simulink model "stepchange_timevarying_change_pure_dual"  (R2022b)
settings: Solver=VariableStepAuto  StartTime=0.0  StopTime=8  MaxStep=0.001  RelTol=1e-3
values from neighbouring files (symbols this model uses):
  A = [eye(N),     -LoadZ^-1,   B; zeros(BN,N),  R_l^-1*B',   eye(BN); zeros(1,N),  zeros(1,N),   V_r'*B ]    [stepchange_timevarying_change_initial_document.m]
  A_r = kron(diag(r),eye(N+BN+1))    [stepchange_timevarying_change_initial_document.m]
  alpha_u = [1.1    1.4    1.8    1.1           1.1    1.9    1.9    1.2           1.3    1.4    1.8    0.6           1.8    2.1    1.5    0.9]'    [stepchange_timevarying_change_initial_document.m]
  alpha_V = [0.7    0.6    0.8    0.9           0.7    1.2    0.8    1.24           0.3    0.3    0.0    1.70           1.0    0.5    1.1    1.0]'    [stepchange_timevarying_change_initial_document.m]
  alpha_w = 0.8    [stepchange_timevarying_change_initial_document.m]
  BN = size(Line1,1)/2    [stepchange_timevarying_change_initial_document.m]
  box_gain = 100    [stepchange_timevarying_change_initial_document.m]
  changerate = 3    [stepchange_timevarying_change_initial_document.m]
  changetime = 5    [stepchange_timevarying_change_initial_document.m]
  changevariance = 0.1    [stepchange_timevarying_change_initial_document.m]
  constraint_gain = 200    [stepchange_timevarying_change_initial_document.m]
  Dw = 0.01    [stepchange_timevarying_change_initial_document.m]
  epsilon = 2    [stepchange_timevarying_change_initial_document.m]
  F_x = blkdiag(diag(r)*diag(alpha_I)+diag(r)*pr*diag(V_r),diag(r)*diag(alpha_V),F_x_I)    [stepchange_timevarying_change_initial_document.m]
  kappa = 10    [stepchange_timevarying_change_initial_document.m]
  l = 2.5    [stepchange_timevarying_change_initial_document.m]
  lambda_I_low_ini = zeros(BN,1)    [stepchange_timevarying_change_initial_document.m]
  lambda_I_up_ini = zeros(BN,1)    [stepchange_timevarying_change_initial_document.m]
  lambda_ini = zeros(N*(BN+N+1),1)    [stepchange_timevarying_change_initial_document.m]
  lambda_v_low_ini = zeros(N,1)    [stepchange_timevarying_change_initial_document.m]
  lambda_v_up_ini = zeros(N,1)    [stepchange_timevarying_change_initial_document.m]
  Lap = 1000*(Degree-Adjacent)    [stepchange_timevarying_change_initial_document.m]
  Lap_BN_plus_N = kron(Lap,eye(BN+N+1))    [stepchange_timevarying_change_initial_document.m]
  Lineconstrants = 10*ones(BN,1)    [stepchange_timevarying_change_initial_document.m]
  Lineindex = zeros(BN,4)    [stepchange_timevarying_change_initial_document.m]
  LoadI = [30.0;15.0;30.0;26.0;         18.9;22.8;29.6;32.1;         22.6;27.6;16.5;19.9;         26.5;19.4;22.7;24.9]    [stepchange_timevarying_change_initial_document.m]
  LoadIchange = [30.0;15.0;30.0;26.0;         18.9;22.8;29.6;32.1;         22.6;27.6;16.5;19.9;         26.5;19.4;22.7;24.9]+3*ones(N,1)    [stepchange_timevarying_change_initial_document.m]
  LoadIchangeno = 3    [stepchange_timevarying_change_initial_document.m]
  LoadZ = diag([16.7;50.0;16.7;20.0;              25.0;16.0;14.2;29.4;              18.5;19.6;22.6;25.6;              23.4;26.4;25.2;33.7])    [stepchange_timevarying_change_initial_document.m]
  LoadZchange = diag([16.7;50.0;16.7;20.0;              25.0;16.0;14.2;29.4;              18.5;19.6;22.6;25.6;              23.4;26.4;25.2;33.7])+3*diag(ones(N,1))    [stepchange_timevarying_change_initial_document.m]
  LoadZchangeno = 3    [stepchange_timevarying_change_initial_document.m]
  localcons_gain = 10    [stepchange_timevarying_change_initial_document.m]
  N = 16    [stepchange_timevarying_change_initial_document.m]
  NCLN = zeros(N,1)    [stepchange_timevarying_change_initial_document.m]
  nu_ini = [-0.00758212493845042	-0.0182492317603708	0.00714905390846842	0.0186908981861182          -0.00758212493845042	-0.0182492317603708	0.00714905390846842	0.0186908981861182          -0.00758212493845042	-0.0182492317603708	0.00714905390846842	0.0186908981861182          -0.00758212493845042	-0.0182492317603708	0.00714905390846842	0.0186908981861182]'    [stepchange_timevarying_change_initial_document.m]
  pr = 0.005    [stepchange_timevarying_change_initial_document.m]
  r = [1.06 1.03 1.05 1.04     1.02 1.03 1.04 1.01     1.03 1.04 1.06 1.07     1.01 1.03 1.04 1.02]    [stepchange_timevarying_change_initial_document.m]
  R = diag([2.0 1.8 1.6 1.5          2.2 1.9 2.6 2.8          1.7 1.9 2.4 2.3          2.6 2.1 2.0 1.9]*10^-2)    [stepchange_timevarying_change_initial_document.m]
  s_A = zeros(N*(N+BN+1),1)    [stepchange_timevarying_change_initial_document.m]
  sigma_ini = zeros(N,1)    [stepchange_timevarying_change_initial_document.m]
  theta_ini = zeros(N*(BN+N+1),1)    [stepchange_timevarying_change_initial_document.m]
  u_ini = [378.9289  380.4146  379.7396  379.2243  380.1955  381.1042         379.9247  379.8974  380.0252  380.4045  379.6763  379.8341         380.1194  380.5682  379.3881  379.9696]'    [stepchange_timevarying_change_initial_document.m]
  upsilon_ini = [172.552238898892	172.552238898892	172.552238898892	172.552238898892               172.552238898892	172.552238898892	172.552238898892	172.552238898892               172.552238898892	172.552238898892	172.552238898892	172.552238898892               172.552238898892	172.552238898892	172.552238898892	172.552238898892]'    [stepchange_timevarying_change_initial_document.m]
  V_hat_low = (380-3)*ones(N,1)    [stepchange_timevarying_change_initial_document.m]
  V_hat_up = (380+3)*ones(N,1)    [stepchange_timevarying_change_initial_document.m]
  V_r = [380.16  381.31  380.27  380.13       380.12  381.24  380.15  380.35       380.15  381.13  380.09  380.22       380.19  381.26  380.21  380.19]'    [stepchange_timevarying_change_initial_document.m]
  varepsilon = 50    [stepchange_timevarying_change_initial_document.m]
  x_hat_ini = [14.515064754915	3.95935897697232	32.9787419273847	14.9071228299889             37.6257931691129	61.1095883901259	41.4721611959256	33.6364102939300             44.9867290171943	52.8132621486412	28.1355733315040	33.0707668633162             36.6024320622732	49.3936276267038	2.38033527987224	36.4476162672594             378.638597580330	380.343321138855	379.211948658584	379.000752058610              ...(+639 chars)    [stepchange_timevarying_change_initial_document.m]
libraries: fl_lib x204, nesl_utility x101, simulink x2, spspowerguiLib x1
(part 2 of 3)

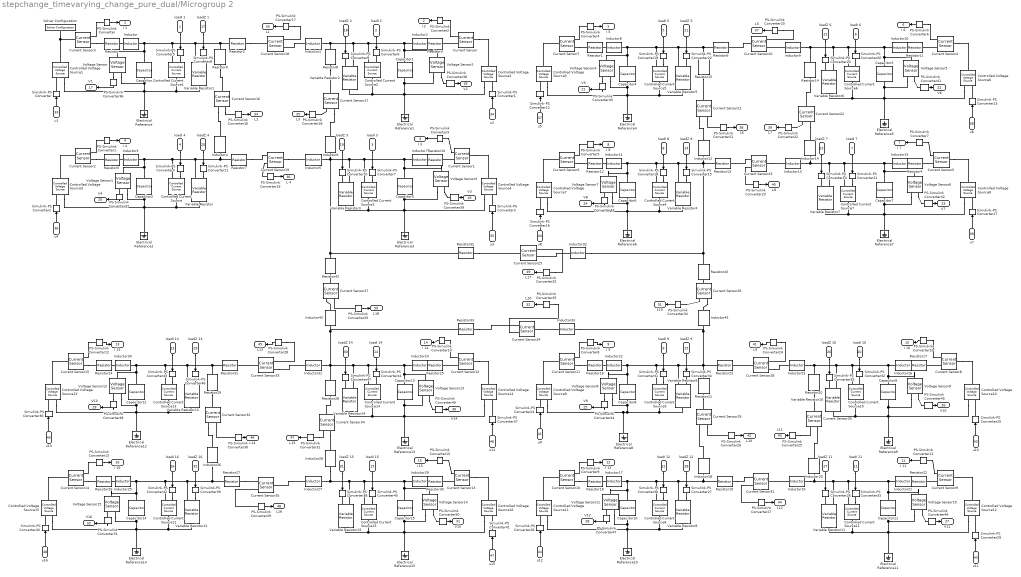
== system stepchange_timevarying_change_pure_dual/Microgroup 2 ==
  loadI 1 : Inport
  loadI 2 : Inport  Port=2
  loadI 3 : Inport  Port=3
  loadI 4 : Inport  Port=4
  loadI 5 : Inport  Port=5
  loadI 6 : Inport  Port=6
  loadI 7 : Inport  Port=7
  loadI 8 : Inport  Port=8
  loadI 9 : Inport  Port=9
  loadI 10 : Inport  Port=10
  loadI 11 : Inport  Port=11
  loadI 12 : Inport  Port=12
  loadI 13 : Inport  Port=13
  loadI 14 : Inport  Port=14
  loadI 15 : Inport  Port=15
  loadI 16 : Inport  Port=16
  loadZ 1 : Inport  Port=17
  loadZ 2 : Inport  Port=18
  loadZ 3 : Inport  Port=19
  loadZ 4 : Inport  Port=20
  loadZ 5 : Inport  Port=21
  loadZ 6 : Inport  Port=22
  loadZ 7 : Inport  Port=23
  loadZ 8 : Inport  Port=24
  loadZ 9 : Inport  Port=25
  loadZ 10 : Inport  Port=26
  loadZ 11 : Inport  Port=27
  loadZ 12 : Inport  Port=28
  loadZ 13 : Inport  Port=29
  loadZ 14 : Inport  Port=30
  loadZ 15 : Inport  Port=31
  loadZ 16 : Inport  Port=32
  u1 : Inport  Port=33
  u2 : Inport  Port=34
  u3 : Inport  Port=35
  u4 : Inport  Port=36
  u5 : Inport  Port=37
  u6 : Inport  Port=38
  u7 : Inport  Port=39
  u8 : Inport  Port=40
  u9 : Inport  Port=41
  u10 : Inport  Port=42
  u11 : Inport  Port=43
  u12 : Inport  Port=44
  u13 : Inport  Port=45
  u14 : Inport  Port=46
  u15 : Inport  Port=47
  u16 : Inport  Port=48
  Capacitor : fl_lib/Electrical/Electrical Elements/Capacitor  c=0.0022 F  r=0 Ohm  g=0 1/Ohm  i_specify=off  i_priority=None  i=0 A  i_nominal_specify=off  i_nominal_unit=A  i_nominal_value=1  v_specify=off  v_priority=None  v=0 V  v_nominal_specify=off  v_nominal_unit=V  v_nominal_value=1  vc_specify=off  vc_priority=High  vc=0 V  vc_nominal_specify=off  vc_nominal_unit=V  vc_nominal_value=1
  Capacitor{1,10,12..13} (4 alike) : fl_lib/Electrical/Electrical Elements/Capacitor  c=0.0019 F  r=0 Ohm  g=0 1/Ohm  i_specify=off  i_priority=None  i=0 A  i_nominal_specify=off  i_nominal_unit=A  i_nominal_value=1  v_specify=off  v_priority=None  v=0 V  v_nominal_specify=off  v_nominal_unit=V  v_nominal_value=1  vc_specify=off  vc_priority=High  vc=0 V  vc_nominal_specify=off  vc_nominal_unit=V  vc_nominal_value=1
  Capacitor11 : fl_lib/Electrical/Electrical Elements/Capacitor  c=0.0026 F  r=0 Ohm  g=0 1/Ohm  i_specify=off  i_priority=None  i=0 A  i_nominal_specify=off  i_nominal_unit=A  i_nominal_value=1  v_specify=off  v_priority=None  v=0 V  v_nominal_specify=off  v_nominal_unit=V  v_nominal_value=1  vc_specify=off  vc_priority=High  vc=0 V  vc_nominal_specify=off  vc_nominal_unit=V  vc_nominal_value=1
  Capacitor14 : fl_lib/Electrical/Electrical Elements/Capacitor  c=0.0023 F  r=0 Ohm  g=0 1/Ohm  i_specify=off  i_priority=None  i=0 A  i_nominal_specify=off  i_nominal_unit=A  i_nominal_value=1  v_specify=off  v_priority=None  v=0 V  v_nominal_specify=off  v_nominal_unit=V  v_nominal_value=1  vc_specify=off  vc_priority=High  vc=0 V  vc_nominal_specify=off  vc_nominal_unit=V  vc_nominal_value=1
  Capacitor15 : fl_lib/Electrical/Electrical Elements/Capacitor  c=0.0022 F  r=0 Ohm  g=0 1/Ohm  i_specify=off  i_priority=None  i=0 A  i_nominal_specify=off  i_nominal_unit=A  i_nominal_value=1  v_specify=off  v_priority=None  v=0 V  v_nominal_specify=off  v_nominal_unit=V  v_nominal_value=1  vc_specify=off  vc_priority=High  vc=0 V  vc_nominal_specify=off  vc_nominal_unit=V  vc_nominal_value=1
  Capacitor2 : fl_lib/Electrical/Electrical Elements/Capacitor  c=0.0017 F  r=0 Ohm  g=0 1/Ohm  i_specify=off  i_priority=None  i=0 A  i_nominal_specify=off  i_nominal_unit=A  i_nominal_value=1  v_specify=off  v_priority=None  v=0 V  v_nominal_specify=off  v_nominal_unit=V  v_nominal_value=1  vc_specify=off  vc_priority=High  vc=0 V  vc_nominal_specify=off  vc_nominal_unit=V  vc_nominal_value=1
  Capacitor3 : fl_lib/Electrical/Electrical Elements/Capacitor  c=0.0025 F  r=0 Ohm  g=0 1/Ohm  i_specify=off  i_priority=None  i=0 A  i_nominal_specify=off  i_nominal_unit=A  i_nominal_value=1  v_specify=off  v_priority=None  v=0 V  v_nominal_specify=off  v_nominal_unit=V  v_nominal_value=1  vc_specify=off  vc_priority=High  vc=0 V  vc_nominal_specify=off  vc_nominal_unit=V  vc_nominal_value=1
  Capacitor4 : fl_lib/Electrical/Electrical Elements/Capacitor  c=0.0018 F  r=0 Ohm  g=0 1/Ohm  i_specify=off  i_priority=None  i=0 A  i_nominal_specify=off  i_nominal_unit=A  i_nominal_value=1  v_specify=off  v_priority=None  v=0 V  v_nominal_specify=off  v_nominal_unit=V  v_nominal_value=1  vc_specify=off  vc_priority=High  vc=0 V  vc_nominal_specify=off  vc_nominal_unit=V  vc_nominal_value=1
  Capacitor5 : fl_lib/Electrical/Electrical Elements/Capacitor  c=0.0022 F  r=0 Ohm  g=0 1/Ohm  i_specify=off  i_priority=None  i=0 A  i_nominal_specify=off  i_nominal_unit=A  i_nominal_value=1  v_specify=off  v_priority=None  v=0 V  v_nominal_specify=off  v_nominal_unit=V  v_nominal_value=1  vc_specify=off  vc_priority=High  vc=0 V  vc_nominal_specify=off  vc_nominal_unit=V  vc_nominal_value=1
  Capacitor6 : fl_lib/Electrical/Electrical Elements/Capacitor  c=0.0031 F  r=0 Ohm  g=0 1/Ohm  i_specify=off  i_priority=None  i=0 A  i_nominal_specify=off  i_nominal_unit=A  i_nominal_value=1  v_specify=off  v_priority=None  v=0 V  v_nominal_specify=off  v_nominal_unit=V  v_nominal_value=1  vc_specify=off  vc_priority=High  vc=0 V  vc_nominal_specify=off  vc_nominal_unit=V  vc_nominal_value=1
  Capacitor7 : fl_lib/Electrical/Electrical Elements/Capacitor  c=0.0029 F  r=0 Ohm  g=0 1/Ohm  i_specify=off  i_priority=None  i=0 A  i_nominal_specify=off  i_nominal_unit=A  i_nominal_value=1  v_specify=off  v_priority=None  v=0 V  v_nominal_specify=off  v_nominal_unit=V  v_nominal_value=1  vc_specify=off  vc_priority=High  vc=0 V  vc_nominal_specify=off  vc_nominal_unit=V  vc_nominal_value=1
  Capacitor8 : fl_lib/Electrical/Electrical Elements/Capacitor  c=0.0017 F  r=0 Ohm  g=0 1/Ohm  i_specify=off  i_priority=None  i=0 A  i_nominal_specify=off  i_nominal_unit=A  i_nominal_value=1  v_specify=off  v_priority=None  v=0 V  v_nominal_specify=off  v_nominal_unit=V  v_nominal_value=1  vc_specify=off  vc_priority=High  vc=0 V  vc_nominal_specify=off  vc_nominal_unit=V  vc_nominal_value=1
  Capacitor9 : fl_lib/Electrical/Electrical Elements/Capacitor  c=0.0025 F  r=0 Ohm  g=0 1/Ohm  i_specify=off  i_priority=None  i=0 A  i_nominal_specify=off  i_nominal_unit=A  i_nominal_value=1  v_specify=off  v_priority=None  v=0 V  v_nominal_specify=off  v_nominal_unit=V  v_nominal_value=1  vc_specify=off  vc_priority=High  vc=0 V  vc_nominal_specify=off  vc_nominal_unit=V  vc_nominal_value=1
  Controlled Current Source{,1..15} (16 alike) : fl_lib/Electrical/Electrical Sources/Controlled Current Source
  Controlled Voltage Source{1..16} (16 alike) : fl_lib/Electrical/Electrical Sources/Controlled Voltage Source
  Current Sensor{,1..35} (36 alike) : fl_lib/Electrical/Electrical Sensors/Current Sensor
  Electrical Reference{,1..15} (16 alike) : fl_lib/Electrical/Electrical Elements/Electrical Reference
  Inductor : fl_lib/Electrical/Electrical Elements/Inductor  l=0.0018 H  r=0 Ohm  g=1e-9 1/Ohm  i_specify=off  i_priority=None  i=0 A  i_nominal_specify=off  i_nominal_unit=A  i_nominal_value=1  v_specify=off  v_priority=None  v=0 V  v_nominal_specify=off  v_nominal_unit=V  v_nominal_value=1  i_L_specify=off  i_L_priority=High  i_L=0 A  i_L_nominal_specify=off  i_L_nominal_unit=A  i_L_nominal_value=1
  Inductor1 : fl_lib/Electrical/Electrical Elements/Inductor  l=2.1000e-06 H  r=0 Ohm  g=1e-9 1/Ohm  i_specify=off  i_priority=None  i=0 A  i_nominal_specify=off  i_nominal_unit=A  i_nominal_value=1  v_specify=off  v_priority=None  v=0 V  v_nominal_specify=off  v_nominal_unit=V  v_nominal_value=1  i_L_specify=off  i_L_priority=High  i_L=0 A  i_L_nominal_specify=off  i_L_nominal_unit=A  i_L_nominal_value=1
  Inductor10 : fl_lib/Electrical/Electrical Elements/Inductor  l=0.0023 H  r=0 Ohm  g=1e-9 1/Ohm  i_specify=off  i_priority=None  i=0 A  i_nominal_specify=off  i_nominal_unit=A  i_nominal_value=1  v_specify=off  v_priority=None  v=0 V  v_nominal_specify=off  v_nominal_unit=V  v_nominal_value=1  i_L_specify=off  i_L_priority=High  i_L=0 A  i_L_nominal_specify=off  i_L_nominal_unit=A  i_L_nominal_value=1
  Inductor11 : fl_lib/Electrical/Electrical Elements/Inductor  l=0.0025 H  r=0 Ohm  g=1e-9 1/Ohm  i_specify=off  i_priority=None  i=0 A  i_nominal_specify=off  i_nominal_unit=A  i_nominal_value=1  v_specify=off  v_priority=None  v=0 V  v_nominal_specify=off  v_nominal_unit=V  v_nominal_value=1  i_L_specify=off  i_L_priority=High  i_L=0 A  i_L_nominal_specify=off  i_L_nominal_unit=A  i_L_nominal_value=1
  Inductor12 : fl_lib/Electrical/Electrical Elements/Inductor  l=2.6000e-06 H  r=0 Ohm  g=1e-9 1/Ohm  i_specify=off  i_priority=None  i=0 A  i_nominal_specify=off  i_nominal_unit=A  i_nominal_value=1  v_specify=off  v_priority=None  v=0 V  v_nominal_specify=off  v_nominal_unit=V  v_nominal_value=1  i_L_specify=off  i_L_priority=High  i_L=0 A  i_L_nominal_specify=off  i_L_nominal_unit=A  i_L_nominal_value=1
  Inductor13 : fl_lib/Electrical/Electrical Elements/Inductor  l=1.9000e-06 H  r=0 Ohm  g=1e-9 1/Ohm  i_specify=off  i_priority=None  i=0 A  i_nominal_specify=off  i_nominal_unit=A  i_nominal_value=1  v_specify=off  v_priority=None  v=0 V  v_nominal_specify=off  v_nominal_unit=V  v_nominal_value=1  i_L_specify=off  i_L_priority=High  i_L=0 A  i_L_nominal_specify=off  i_L_nominal_unit=A  i_L_nominal_value=1
  Inductor14 : fl_lib/Electrical/Electrical Elements/Inductor  l=2.0000e-06 H  r=0 Ohm  g=1e-9 1/Ohm  i_specify=off  i_priority=None  i=0 A  i_nominal_specify=off  i_nominal_unit=A  i_nominal_value=1  v_specify=off  v_priority=None  v=0 V  v_nominal_specify=off  v_nominal_unit=V  v_nominal_value=1  i_L_specify=off  i_L_priority=High  i_L=0 A  i_L_nominal_specify=off  i_L_nominal_unit=A  i_L_nominal_value=1
  Inductor15 : fl_lib/Electrical/Electrical Elements/Inductor  l=0.0019 H  r=0 Ohm  g=1e-9 1/Ohm  i_specify=off  i_priority=None  i=0 A  i_nominal_specify=off  i_nominal_unit=A  i_nominal_value=1  v_specify=off  v_priority=None  v=0 V  v_nominal_specify=off  v_nominal_unit=V  v_nominal_value=1  i_L_specify=off  i_L_priority=High  i_L=0 A  i_L_nominal_specify=off  i_L_nominal_unit=A  i_L_nominal_value=1
  Inductor16 : fl_lib/Electrical/Electrical Elements/Inductor  l=0.0022 H  r=0 Ohm  g=1e-9 1/Ohm  i_specify=off  i_priority=None  i=0 A  i_nominal_specify=off  i_nominal_unit=A  i_nominal_value=1  v_specify=off  v_priority=None  v=0 V  v_nominal_specify=off  v_nominal_unit=V  v_nominal_value=1  i_L_specify=off  i_L_priority=High  i_L=0 A  i_L_nominal_specify=off  i_L_nominal_unit=A  i_L_nominal_value=1
  Inductor17 : fl_lib/Electrical/Electrical Elements/Inductor  l=0.0029 H  r=0 Ohm  g=1e-9 1/Ohm  i_specify=off  i_priority=None  i=0 A  i_nominal_specify=off  i_nominal_unit=A  i_nominal_value=1  v_specify=off  v_priority=None  v=0 V  v_nominal_specify=off  v_nominal_unit=V  v_nominal_value=1  i_L_specify=off  i_L_priority=High  i_L=0 A  i_L_nominal_specify=off  i_L_nominal_unit=A  i_L_nominal_value=1
  Inductor18 : fl_lib/Electrical/Electrical Elements/Inductor  l=2.5000e-06 H  r=0 Ohm  g=1e-9 1/Ohm  i_specify=off  i_priority=None  i=0 A  i_nominal_specify=off  i_nominal_unit=A  i_nominal_value=1  v_specify=off  v_priority=None  v=0 V  v_nominal_specify=off  v_nominal_unit=V  v_nominal_value=1  i_L_specify=off  i_L_priority=High  i_L=0 A  i_L_nominal_specify=off  i_L_nominal_unit=A  i_L_nominal_value=1
  Inductor19 : fl_lib/Electrical/Electrical Elements/Inductor  l=2.4000e-06 H  r=0 Ohm  g=1e-9 1/Ohm  i_specify=off  i_priority=None  i=0 A  i_nominal_specify=off  i_nominal_unit=A  i_nominal_value=1  v_specify=off  v_priority=None  v=0 V  v_nominal_specify=off  v_nominal_unit=V  v_nominal_value=1  i_L_specify=off  i_L_priority=High  i_L=0 A  i_L_nominal_specify=off  i_L_nominal_unit=A  i_L_nominal_value=1
  Inductor2 : fl_lib/Electrical/Electrical Elements/Inductor  l=0.0020 H  r=0 Ohm  g=1e-9 1/Ohm  i_specify=off  i_priority=None  i=0 A  i_nominal_specify=off  i_nominal_unit=A  i_nominal_value=1  v_specify=off  v_priority=None  v=0 V  v_nominal_specify=off  v_nominal_unit=V  v_nominal_value=1  i_L_specify=off  i_L_priority=High  i_L=0 A  i_L_nominal_specify=off  i_L_nominal_unit=A  i_L_nominal_value=1
  Inductor20 : fl_lib/Electrical/Electrical Elements/Inductor  l=2.8000e-06 H  r=0 Ohm  g=1e-9 1/Ohm  i_specify=off  i_priority=None  i=0 A  i_nominal_specify=off  i_nominal_unit=A  i_nominal_value=1  v_specify=off  v_priority=None  v=0 V  v_nominal_specify=off  v_nominal_unit=V  v_nominal_value=1  i_L_specify=off  i_L_priority=High  i_L=0 A  i_L_nominal_specify=off  i_L_nominal_unit=A  i_L_nominal_value=1
  Inductor21 : fl_lib/Electrical/Electrical Elements/Inductor  l=0.0023 H  r=0 Ohm  g=1e-9 1/Ohm  i_specify=off  i_priority=None  i=0 A  i_nominal_specify=off  i_nominal_unit=A  i_nominal_value=1  v_specify=off  v_priority=None  v=0 V  v_nominal_specify=off  v_nominal_unit=V  v_nominal_value=1  i_L_specify=off  i_L_priority=High  i_L=0 A  i_L_nominal_specify=off  i_L_nominal_unit=A  i_L_nominal_value=1
  Inductor22 : fl_lib/Electrical/Electrical Elements/Inductor  l=0.0017 H  r=0 Ohm  g=1e-9 1/Ohm  i_specify=off  i_priority=None  i=0 A  i_nominal_specify=off  i_nominal_unit=A  i_nominal_value=1  v_specify=off  v_priority=None  v=0 V  v_nominal_specify=off  v_nominal_unit=V  v_nominal_value=1  i_L_specify=off  i_L_priority=High  i_L=0 A  i_L_nominal_specify=off  i_L_nominal_unit=A  i_L_nominal_value=1
  Inductor{9,23,31,42} (4 alike) : fl_lib/Electrical/Electrical Elements/Inductor  l=2.3000e-06 H  r=0 Ohm  g=1e-9 1/Ohm  i_specify=off  i_priority=None  i=0 A  i_nominal_specify=off  i_nominal_unit=A  i_nominal_value=1  v_specify=off  v_priority=None  v=0 V  v_nominal_specify=off  v_nominal_unit=V  v_nominal_value=1  i_L_specify=off  i_L_priority=High  i_L=0 A  i_L_nominal_specify=off  i_L_nominal_unit=A  i_L_nominal_value=1
  Inductor24 : fl_lib/Electrical/Electrical Elements/Inductor  l=0.0025 H  r=0 Ohm  g=1e-9 1/Ohm  i_specify=off  i_priority=None  i=0 A  i_nominal_specify=off  i_nominal_unit=A  i_nominal_value=1  v_specify=off  v_priority=None  v=0 V  v_nominal_specify=off  v_nominal_unit=V  v_nominal_value=1  i_L_specify=off  i_L_priority=High  i_L=0 A  i_L_nominal_specify=off  i_L_nominal_unit=A  i_L_nominal_value=1
  Inductor25 : fl_lib/Electrical/Electrical Elements/Inductor  l=0.0030 H  r=0 Ohm  g=1e-9 1/Ohm  i_specify=off  i_priority=None  i=0 A  i_nominal_specify=off  i_nominal_unit=A  i_nominal_value=1  v_specify=off  v_priority=None  v=0 V  v_nominal_specify=off  v_nominal_unit=V  v_nominal_value=1  i_L_specify=off  i_L_priority=High  i_L=0 A  i_L_nominal_specify=off  i_L_nominal_unit=A  i_L_nominal_value=1
  Inductor26 : fl_lib/Electrical/Electrical Elements/Inductor  l=2.5000e-06 H  r=0 Ohm  g=1e-9 1/Ohm  i_specify=off  i_priority=None  i=0 A  i_nominal_specify=off  i_nominal_unit=A  i_nominal_value=1  v_specify=off  v_priority=None  v=0 V  v_nominal_specify=off  v_nominal_unit=V  v_nominal_value=1  i_L_specify=off  i_L_priority=High  i_L=0 A  i_L_nominal_specify=off  i_L_nominal_unit=A  i_L_nominal_value=1
  Inductor27 : fl_lib/Electrical/Electrical Elements/Inductor  l=2.4000e-06 H  r=0 Ohm  g=1e-9 1/Ohm  i_specify=off  i_priority=None  i=0 A  i_nominal_specify=off  i_nominal_unit=A  i_nominal_value=1  v_specify=off  v_priority=None  v=0 V  v_nominal_specify=off  v_nominal_unit=V  v_nominal_value=1  i_L_specify=off  i_L_priority=High  i_L=0 A  i_L_nominal_specify=off  i_L_nominal_unit=A  i_L_nominal_value=1
  Inductor28 : fl_lib/Electrical/Electrical Elements/Inductor  l=2.6000e-06 H  r=0 Ohm  g=1e-9 1/Ohm  i_specify=off  i_priority=None  i=0 A  i_nominal_specify=off  i_nominal_unit=A  i_nominal_value=1  v_specify=off  v_priority=None  v=0 V  v_nominal_specify=off  v_nominal_unit=V  v_nominal_value=1  i_L_specify=off  i_L_priority=High  i_L=0 A  i_L_nominal_specify=off  i_L_nominal_unit=A  i_L_nominal_value=1
  Inductor29 : fl_lib/Electrical/Electrical Elements/Inductor  l=0.0019 H  r=0 Ohm  g=1e-9 1/Ohm  i_specify=off  i_priority=None  i=0 A  i_nominal_specify=off  i_nominal_unit=A  i_nominal_value=1  v_specify=off  v_priority=None  v=0 V  v_nominal_specify=off  v_nominal_unit=V  v_nominal_value=1  i_L_specify=off  i_L_priority=High  i_L=0 A  i_L_nominal_specify=off  i_L_nominal_unit=A  i_L_nominal_value=1
  Inductor3 : fl_lib/Electrical/Electrical Elements/Inductor  l=0.0022 H  r=0 Ohm  g=1e-9 1/Ohm  i_specify=off  i_priority=None  i=0 A  i_nominal_specify=off  i_nominal_unit=A  i_nominal_value=1  v_specify=off  v_priority=None  v=0 V  v_nominal_specify=off  v_nominal_unit=V  v_nominal_value=1  i_L_specify=off  i_L_priority=High  i_L=0 A  i_L_nominal_specify=off  i_L_nominal_unit=A  i_L_nominal_value=1
  Inductor30 : fl_lib/Electrical/Electrical Elements/Inductor  l=0.0023 H  r=0 Ohm  g=1e-9 1/Ohm  i_specify=off  i_priority=None  i=0 A  i_nominal_specify=off  i_nominal_unit=A  i_nominal_value=1  v_specify=off  v_priority=None  v=0 V  v_nominal_specify=off  v_nominal_unit=V  v_nominal_value=1  i_L_specify=off  i_L_priority=High  i_L=0 A  i_L_nominal_specify=off  i_L_nominal_unit=A  i_L_nominal_value=1
  Inductor32 : fl_lib/Electrical/Electrical Elements/Inductor  l=2.1000e-06 H  r=0 Ohm  g=1e-9 1/Ohm  i_specify=off  i_priority=None  i=0 A  i_nominal_specify=off  i_nominal_unit=A  i_nominal_value=1  v_specify=off  v_priority=None  v=0 V  v_nominal_specify=off  v_nominal_unit=V  v_nominal_value=1  i_L_specify=off  i_L_priority=High  i_L=0 A  i_L_nominal_specify=off  i_L_nominal_unit=A  i_L_nominal_value=1
  Inductor33 : fl_lib/Electrical/Electrical Elements/Inductor  l=2.6000e-06 H  r=0 Ohm  g=1e-9 1/Ohm  i_specify=off  i_priority=None  i=0 A  i_nominal_specify=off  i_nominal_unit=A  i_nominal_value=1  v_specify=off  v_priority=None  v=0 V  v_nominal_specify=off  v_nominal_unit=V  v_nominal_value=1  i_L_specify=off  i_L_priority=High  i_L=0 A  i_L_nominal_specify=off  i_L_nominal_unit=A  i_L_nominal_value=1
  Inductor4 : fl_lib/Electrical/Electrical Elements/Inductor  l=2.0000e-06 H  r=0 Ohm  g=1e-9 1/Ohm  i_specify=off  i_priority=None  i=0 A  i_nominal_specify=off  i_nominal_unit=A  i_nominal_value=1  v_specify=off  v_priority=None  v=0 V  v_nominal_specify=off  v_nominal_unit=V  v_nominal_value=1  i_L_specify=off  i_L_priority=High  i_L=0 A  i_L_nominal_specify=off  i_L_nominal_unit=A  i_L_nominal_value=1
  Inductor43 : fl_lib/Electrical/Electrical Elements/Inductor  l=2.5000e-06 H  r=0 Ohm  g=1e-9 1/Ohm  i_specify=off  i_priority=None  i=0 A  i_nominal_specify=off  i_nominal_unit=A  i_nominal_value=1  v_specify=off  v_priority=None  v=0 V  v_nominal_specify=off  v_nominal_unit=V  v_nominal_value=1  i_L_specify=off  i_L_priority=High  i_L=0 A  i_L_nominal_specify=off  i_L_nominal_unit=A  i_L_nominal_value=1
  Inductor5 : fl_lib/Electrical/Electrical Elements/Inductor  l=2.2000e-06 H  r=0 Ohm  g=1e-9 1/Ohm  i_specify=off  i_priority=None  i=0 A  i_nominal_specify=off  i_nominal_unit=A  i_nominal_value=1  v_specify=off  v_priority=None  v=0 V  v_nominal_specify=off  v_nominal_unit=V  v_nominal_value=1  i_L_specify=off  i_L_priority=High  i_L=0 A  i_L_nominal_specify=off  i_L_nominal_unit=A  i_L_nominal_value=1
  Inductor6 : fl_lib/Electrical/Electrical Elements/Inductor  l=3.0000e-06 H  r=0 Ohm  g=1e-9 1/Ohm  i_specify=off  i_priority=None  i=0 A  i_nominal_specify=off  i_nominal_unit=A  i_nominal_value=1  v_specify=off  v_priority=None  v=0 V  v_nominal_specify=off  v_nominal_unit=V  v_nominal_value=1  i_L_specify=off  i_L_priority=High  i_L=0 A  i_L_nominal_specify=off  i_L_nominal_unit=A  i_L_nominal_value=1
  Inductor7 : fl_lib/Electrical/Electrical Elements/Inductor  l=0.0030 H  r=0 Ohm  g=1e-9 1/Ohm  i_specify=off  i_priority=None  i=0 A  i_nominal_specify=off  i_nominal_unit=A  i_nominal_value=1  v_specify=off  v_priority=None  v=0 V  v_nominal_specify=off  v_nominal_unit=V  v_nominal_value=1  i_L_specify=off  i_L_priority=High  i_L=0 A  i_L_nominal_specify=off  i_L_nominal_unit=A  i_L_nominal_value=1
  Inductor8 : fl_lib/Electrical/Electrical Elements/Inductor  l=0.0022 H  r=0 Ohm  g=1e-9 1/Ohm  i_specify=off  i_priority=None  i=0 A  i_nominal_specify=off  i_nominal_unit=A  i_nominal_value=1  v_specify=off  v_priority=None  v=0 V  v_nominal_specify=off  v_nominal_unit=V  v_nominal_value=1  i_L_specify=off  i_L_priority=High  i_L=0 A  i_L_nominal_specify=off  i_L_nominal_unit=A  i_L_nominal_value=1
  PS-Simulink Converter{,1..51} (52 alike) : nesl_utility/PS-Simulink Converter  PhysicalDomain=network_engine_domain  SubClassName=ps_output  LeftPortType=input  RightPortType=output  PseudoPeriodic=off  Frequencies=[]  VectorFormat=inherit  Unit=inherit  AffineConversion=off
  Resistor : fl_lib/Electrical/Electrical Elements/Resistor  R=0.020+alpha_w Ohm  i_specify=off  i_priority=None  i=0 A  i_nominal_specify=off  i_nominal_unit=A  i_nominal_value=1  v_specify=off  v_priority=None  v=0 V  v_nominal_specify=off  v_nominal_unit=V  v_nominal_value=1
  Resistor1 : fl_lib/Electrical/Electrical Elements/Resistor  R=0.0220+alpha_w Ohm  i_specify=off  i_priority=None  i=0 A  i_nominal_specify=off  i_nominal_unit=A  i_nominal_value=1  v_specify=off  v_priority=None  v=0 V  v_nominal_specify=off  v_nominal_unit=V  v_nominal_value=1
  Resistor10 : fl_lib/Electrical/Electrical Elements/Resistor  R=0.0160+alpha_w Ohm  i_specify=off  i_priority=None  i=0 A  i_nominal_specify=off  i_nominal_unit=A  i_nominal_value=1  v_specify=off  v_priority=None  v=0 V  v_nominal_specify=off  v_nominal_unit=V  v_nominal_value=1
  Resistor11 : fl_lib/Electrical/Electrical Elements/Resistor  R=0.019+alpha_w Ohm  i_specify=off  i_priority=None  i=0 A  i_nominal_specify=off  i_nominal_unit=A  i_nominal_value=1  v_specify=off  v_priority=None  v=0 V  v_nominal_specify=off  v_nominal_unit=V  v_nominal_value=1
  Resistor12 : fl_lib/Electrical/Electrical Elements/Resistor  R=0.028+alpha_w Ohm  i_specify=off  i_priority=None  i=0 A  i_nominal_specify=off  i_nominal_unit=A  i_nominal_value=1  v_specify=off  v_priority=None  v=0 V  v_nominal_specify=off  v_nominal_unit=V  v_nominal_value=1
  Resistor{7,13,20,42} (4 alike) : fl_lib/Electrical/Electrical Elements/Resistor  R=0.0600 Ohm  i_specify=off  i_priority=None  i=0 A  i_nominal_specify=off  i_nominal_unit=A  i_nominal_value=1  v_specify=off  v_priority=None  v=0 V  v_nominal_specify=off  v_nominal_unit=V  v_nominal_value=1
  Resistor14 : fl_lib/Electrical/Electrical Elements/Resistor  R=0.0500 Ohm  i_specify=off  i_priority=None  i=0 A  i_nominal_specify=off  i_nominal_unit=A  i_nominal_value=1  v_specify=off  v_priority=None  v=0 V  v_nominal_specify=off  v_nominal_unit=V  v_nominal_value=1
  Resistor{6,8,15,23,28,31,33} (7 alike) : fl_lib/Electrical/Electrical Elements/Resistor  R=0.0800 Ohm  i_specify=off  i_priority=None  i=0 A  i_nominal_specify=off  i_nominal_unit=A  i_nominal_value=1  v_specify=off  v_priority=None  v=0 V  v_nominal_specify=off  v_nominal_unit=V  v_nominal_value=1
  Resistor16 : fl_lib/Electrical/Electrical Elements/Resistor  R=0.017+alpha_w Ohm  i_specify=off  i_priority=None  i=0 A  i_nominal_specify=off  i_nominal_unit=A  i_nominal_value=1  v_specify=off  v_priority=None  v=0 V  v_nominal_specify=off  v_nominal_unit=V  v_nominal_value=1
  Resistor17 : fl_lib/Electrical/Electrical Elements/Resistor  R=0.019+alpha_w Ohm  i_specify=off  i_priority=None  i=0 A  i_nominal_specify=off  i_nominal_unit=A  i_nominal_value=1  v_specify=off  v_priority=None  v=0 V  v_nominal_specify=off  v_nominal_unit=V  v_nominal_value=1
  Resistor18 : fl_lib/Electrical/Electrical Elements/Resistor  R=0.023+alpha_w Ohm  i_specify=off  i_priority=None  i=0 A  i_nominal_specify=off  i_nominal_unit=A  i_nominal_value=1  v_specify=off  v_priority=None  v=0 V  v_nominal_specify=off  v_nominal_unit=V  v_nominal_value=1
  Resistor{2,19,21,29,32,43} (6 alike) : fl_lib/Electrical/Electrical Elements/Resistor  R=0.0700 Ohm  i_specify=off  i_priority=None  i=0 A  i_nominal_specify=off  i_nominal_unit=A  i_nominal_value=1  v_specify=off  v_priority=None  v=0 V  v_nominal_specify=off  v_nominal_unit=V  v_nominal_value=1
  Resistor22 : fl_lib/Electrical/Electrical Elements/Resistor  R=0.024+alpha_w Ohm  i_specify=off  i_priority=None  i=0 A  i_nominal_specify=off  i_nominal_unit=A  i_nominal_value=1  v_specify=off  v_priority=None  v=0 V  v_nominal_specify=off  v_nominal_unit=V  v_nominal_value=1
  Resistor24 : fl_lib/Electrical/Electrical Elements/Resistor  R=0.026+alpha_w Ohm  i_specify=off  i_priority=None  i=0 A  i_nominal_specify=off  i_nominal_unit=A  i_nominal_value=1  v_specify=off  v_priority=None  v=0 V  v_nominal_specify=off  v_nominal_unit=V  v_nominal_value=1
  Resistor25 : fl_lib/Electrical/Electrical Elements/Resistor  R=0.021+alpha_w Ohm  i_specify=off  i_priority=None  i=0 A  i_nominal_specify=off  i_nominal_unit=A  i_nominal_value=1  v_specify=off  v_priority=None  v=0 V  v_nominal_specify=off  v_nominal_unit=V  v_nominal_value=1
  Resistor26 : fl_lib/Electrical/Electrical Elements/Resistor  R=0.019+alpha_w Ohm  i_specify=off  i_priority=None  i=0 A  i_nominal_specify=off  i_nominal_unit=A  i_nominal_value=1  v_specify=off  v_priority=None  v=0 V  v_nominal_specify=off  v_nominal_unit=V  v_nominal_value=1
  Resistor27 : fl_lib/Electrical/Electrical Elements/Resistor  R=0.0500 Ohm  i_specify=off  i_priority=None  i=0 A  i_nominal_specify=off  i_nominal_unit=A  i_nominal_value=1  v_specify=off  v_priority=None  v=0 V  v_nominal_specify=off  v_nominal_unit=V  v_nominal_value=1
  Resistor3 : fl_lib/Electrical/Electrical Elements/Resistor  R=0.0180+alpha_w Ohm  i_specify=off  i_priority=None  i=0 A  i_nominal_specify=off  i_nominal_unit=A  i_nominal_value=1  v_specify=off  v_priority=None  v=0 V  v_nominal_specify=off  v_nominal_unit=V  v_nominal_value=1
  Resistor30 : fl_lib/Electrical/Electrical Elements/Resistor  R=0.020+alpha_w Ohm  i_specify=off  i_priority=None  i=0 A  i_nominal_specify=off  i_nominal_unit=A  i_nominal_value=1  v_specify=off  v_priority=None  v=0 V  v_nominal_specify=off  v_nominal_unit=V  v_nominal_value=1
  Resistor4 : fl_lib/Electrical/Electrical Elements/Resistor  R=0.0260+alpha_w Ohm  i_specify=off  i_priority=None  i=0 A  i_nominal_specify=off  i_nominal_unit=A  i_nominal_value=1  v_specify=off  v_priority=None  v=0 V  v_nominal_specify=off  v_nominal_unit=V  v_nominal_value=1
  Resistor5 : fl_lib/Electrical/Electrical Elements/Resistor  R=0.0150+alpha_w Ohm  i_specify=off  i_priority=None  i=0 A  i_nominal_specify=off  i_nominal_unit=A  i_nominal_value=1  v_specify=off  v_priority=None  v=0 V  v_nominal_specify=off  v_nominal_unit=V  v_nominal_value=1
  Resistor9 : fl_lib/Electrical/Electrical Elements/Resistor  R=0.0500 Ohm  i_specify=off  i_priority=None  i=0 A  i_nominal_specify=off  i_nominal_unit=A  i_nominal_value=1  v_specify=off  v_priority=None  v=0 V  v_nominal_specify=off  v_nominal_unit=V  v_nominal_value=1
  Simulink-PS Converter{,1..47} (48 alike) : nesl_utility/Simulink-PS Converter  PhysicalDomain=network_engine_domain  SubClassName=ps_input  LeftPortType=input  RightPortType=output  PseudoPeriodic=off  Frequencies=[]  NoiseDistribution=none  NoiseParameters=[]  Unit=1  AffineConversion=off  FilteringAndDerivatives=provide  SimscapeFilterOrder=1  InputFilterTimeConstant=0.001  UdotUserProvided=0
  Solver Configuration : nesl_utility/Solver Configuration  PhysicalDomain=network_engine_domain  SubClassName=solver  LeftPortType=input  RightPortType=generic  Tones=[]  Harmonics=[]  SimulateNoise=off  Profile=off  UseLocalSampling=off  EnableSwitchedLinearOptims=on  FrequencyDomain=off  UseCCode=off  RelTol=0.001  AbsTol=0.001  MinStep=1e-09  ToWorkspace=off  RevertToSquareIcSolve=off  NumHomotopyIterations=100  PhasorMode=off  PhasorModeNumHarmonics=1  ConsistencySolver=NEWTON_XTOL_AFTER_FTOL  IndexReductionMethod=DerivativeReplacement  DoDC=off  ResidualTolerance=1e-09  ConsistencyTolSource=GLOBAL  ConsistencyAbsTol=0.001  ConsistencyRelTol=0.001  ConsistencyTolFactor=0.001  UseLocalSolver=off  LocalSolverChoice=NE_BACKWARD_EULER_ADVANCER  ResolveIndetEquations=on  FunctionEvalNumThread=1  LocalSolverSampleTime=0.001  DoFixedCost=off  MaxNonlinIter=3  MaxModeIter=2  ComputeImpulses=off  ImpulseIterations=2  LinearAlgebra=Full  LinearAlgebraNumThread=0  EquationFormulation=NE_TIME_EF  DelaysMemoryBudget=1024  AutomaticFiltering=on  FilteringTimeConstant=0.001  PartitionStorageMethod=AS_NEEDED  PartitionMemoryBudget=1024  PartitionMethod=ROBUST
  Variable Resistor{,1..15} (16 alike) : fl_lib/Electrical/Electrical Elements/Variable Resistor  Rmin=0 Ohm  i_specify=off  i_priority=None  i=0 A  i_nominal_specify=off  i_nominal_unit=A  i_nominal_value=1  v_specify=off  v_priority=None  v=0 V  v_nominal_specify=off  v_nominal_unit=V  v_nominal_value=1
  Voltage Sensor{,1..15} (16 alike) : fl_lib/Electrical/Electrical Sensors/Voltage Sensor
  I 1 : Outport
  I 2 : Outport  Port=2
  I 3 : Outport  Port=3
  I 4 : Outport  Port=4
  I 5 : Outport  Port=5
  I 6 : Outport  Port=6
  I 7 : Outport  Port=7
  I 8 : Outport  Port=8
  I 9 : Outport  Port=9
  I 10 : Outport  Port=10
  I 11 : Outport  Port=11
  I 12 : Outport  Port=12
  I 13 : Outport  Port=13
  I 14 : Outport  Port=14
  I 15 : Outport  Port=15
  I 16 : Outport  Port=16
  V1 : Outport  Port=17
  V2 : Outport  Port=18
  V3 : Outport  Port=19
  V4 : Outport  Port=20
  V5 : Outport  Port=21
  V6 : Outport  Port=22
  V7 : Outport  Port=23
  V8 : Outport  Port=24
  V9 : Outport  Port=25
  V10 : Outport  Port=26
  V11 : Outport  Port=27
  V12 : Outport  Port=28
  V13 : Outport  Port=29
  V14 : Outport  Port=30
  V15 : Outport  Port=31
  V16 : Outport  Port=32
  L1 : Outport  Port=33
  "L2 " : Outport  Port=34
  L3 : Outport  Port=35
  L 4 : Outport  Port=36
  L5 : Outport  Port=37
  L6 : Outport  Port=38
  " L7" : Outport  Port=39
  L8 : Outport  Port=40
  L9 : Outport  Port=41
  L10 : Outport  Port=42
  " L11" : Outport  Port=43
  L12 : Outport  Port=44
  L13 : Outport  Port=45
  L14 : Outport  Port=46
  L15 : Outport  Port=47
  L16 : Outport  Port=48
  L17 : Outport  Port=49
  L18 : Outport  Port=50
  L19 : Outport  Port=51
  L20 : Outport  Port=52
  wires:
  u3/1 -> Simulink-PS Converter3/1
  u2/1 -> Simulink-PS Converter1/1
  u4/1 -> Simulink-PS Converter2/1
  loadI 1/1 -> Simulink-PS Converter5/1
  loadI 4/1 -> Simulink-PS Converter4/1
  loadI 2/1 -> Simulink-PS Converter6/1
  loadI 3/1 -> Simulink-PS Converter7/1
  PS-Simulink Converter/1 -> I 1/1
  PS-Simulink Converter2/1 -> I 2/1
  PS-Simulink Converter3/1 -> I 3/1
  PS-Simulink Converter1/1 -> I 4/1
  loadZ 1/1 -> Simulink-PS Converter8/1
  loadZ 2/1 -> Simulink-PS Converter9/1
  loadZ 3/1 -> Simulink-PS Converter10/1
  loadZ 4/1 -> Simulink-PS Converter11/1
  PS-Simulink Converter4/1 -> I 5/1
  loadZ 8/1 -> Simulink-PS Converter15/1
  loadZ 7/1 -> Simulink-PS Converter14/1
  PS-Simulink Converter6/1 -> I 6/1
  u5/1 -> Simulink-PS Converter12/1
  PS-Simulink Converter7/1 -> I 7/1
  loadZ 5/1 -> Simulink-PS Converter22/1
  loadI 8/1 -> Simulink-PS Converter18/1
  loadI 6/1 -> Simulink-PS Converter20/1
  u8/1 -> Simulink-PS Converter16/1
  loadI 5/1 -> Simulink-PS Converter19/1
  PS-Simulink Converter5/1 -> I 8/1
  loadI 7/1 -> Simulink-PS Converter21/1
  loadZ 6/1 -> Simulink-PS Converter23/1
  u7/1 -> Simulink-PS Converter17/1
  u6/1 -> Simulink-PS Converter13/1
  u10/1 -> Simulink-PS Converter25/1
  u11/1 -> Simulink-PS Converter29/1
  loadZ 10/1 -> Simulink-PS Converter35/1
  loadI 10/1 -> Simulink-PS Converter32/1
  loadI 9/1 -> Simulink-PS Converter31/1
  loadI 12/1 -> Simulink-PS Converter30/1
  u12/1 -> Simulink-PS Converter28/1
  loadZ 9/1 -> Simulink-PS Converter34/1
  loadZ 12/1 -> Simulink-PS Converter27/1
  PS-Simulink Converter9/1 -> I 12/1
  u9/1 -> Simulink-PS Converter24/1
  PS-Simulink Converter10/1 -> I 10/1
  PS-Simulink Converter8/1 -> I 9/1
  PS-Simulink Converter11/1 -> I 11/1
  loadZ 11/1 -> Simulink-PS Converter26/1
  loadI 11/1 -> Simulink-PS Converter33/1
  u14/1 -> Simulink-PS Converter37/1
  u15/1 -> Simulink-PS Converter41/1
  loadZ 14/1 -> Simulink-PS Converter47/1
  loadI 14/1 -> Simulink-PS Converter44/1
  loadI 13/1 -> Simulink-PS Converter43/1
  loadI 16/1 -> Simulink-PS Converter42/1
  u16/1 -> Simulink-PS Converter40/1
  loadZ 13/1 -> Simulink-PS Converter46/1
  loadZ 16/1 -> Simulink-PS Converter39/1
  PS-Simulink Converter13/1 -> I 16/1
  u13/1 -> Simulink-PS Converter36/1
  PS-Simulink Converter14/1 -> I 14/1
  PS-Simulink Converter12/1 -> I 13/1
  PS-Simulink Converter15/1 -> I 15/1
  loadZ 15/1 -> Simulink-PS Converter38/1
  loadI 15/1 -> Simulink-PS Converter45/1
  PS-Simulink Converter16/1 -> "L2 "/1
  PS-Simulink Converter17/1 -> L1/1
  PS-Simulink Converter18/1 -> L3/1
  PS-Simulink Converter19/1 -> L 4/1
  PS-Simulink Converter20/1 -> L5/1
  PS-Simulink Converter21/1 -> L6/1
  PS-Simulink Converter22/1 -> " L7"/1
  PS-Simulink Converter23/1 -> L8/1
  PS-Simulink Converter24/1 -> L9/1
  PS-Simulink Converter25/1 -> " L11"/1
  PS-Simulink Converter26/1 -> L10/1
  PS-Simulink Converter27/1 -> L12/1
  PS-Simulink Converter28/1 -> L13/1
  PS-Simulink Converter29/1 -> L16/1
  PS-Simulink Converter30/1 -> L14/1
  PS-Simulink Converter31/1 -> L15/1
  PS-Simulink Converter32/1 -> L17/1
  PS-Simulink Converter33/1 -> L18/1
  PS-Simulink Converter34/1 -> L19/1
  PS-Simulink Converter35/1 -> L20/1
  PS-Simulink Converter36/1 -> V1/1
  PS-Simulink Converter37/1 -> V4/1
  PS-Simulink Converter38/1 -> V2/1
  PS-Simulink Converter39/1 -> V3/1
  PS-Simulink Converter40/1 -> V5/1
  PS-Simulink Converter41/1 -> V6/1
  PS-Simulink Converter42/1 -> V7/1
  PS-Simulink Converter43/1 -> V8/1
  PS-Simulink Converter44/1 -> V9/1
  PS-Simulink Converter45/1 -> V10/1
  PS-Simulink Converter46/1 -> V11/1
  PS-Simulink Converter47/1 -> V12/1
  PS-Simulink Converter48/1 -> V13/1
  PS-Simulink Converter49/1 -> V14/1
  PS-Simulink Converter50/1 -> V15/1
  PS-Simulink Converter51/1 -> V16/1
  u1/1 -> Simulink-PS Converter/1
  connections:
  Capacitor/LConn1 -- Voltage Sensor/LConn1 -- Inductor/RConn1 -- Resistor9/LConn1 -- Resistor2/LConn1 -- Variable Resistor1/LConn2 -- Controlled Current Source1/RConn2
  Controlled Voltage Source3/RConn2 -- Electrical Reference2/LConn1 -- Voltage Sensor1/RConn2 -- Capacitor2/RConn1 -- Variable Resistor/RConn1 -- Controlled Current Source/LConn1
  Inductor2/RConn1 -- Capacitor1/LConn1 -- Voltage Sensor2/LConn1 -- Resistor8/LConn1 -- Inductor1/RConn1 -- Variable Resistor2/LConn2 -- Controlled Current Source2/RConn2
  Inductor3/RConn1 -- Capacitor2/LConn1 -- Voltage Sensor1/LConn1 -- Inductor4/RConn1 -- Resistor7/LConn1 -- Variable Resistor/LConn2 -- Controlled Current Source/RConn2
  Capacitor3/RConn1 -- Voltage Sensor3/RConn2 -- Controlled Voltage Source4/RConn2 -- Electrical Reference3/LConn1 -- Variable Resistor3/RConn1 -- Controlled Current Source3/LConn1
  Resistor3/RConn1 -- Inductor2/LConn1
  Resistor42/RConn1 -- Inductor6/RConn1 -- Inductor5/RConn1 -- Voltage Sensor3/LConn1 -- Capacitor3/LConn1 -- Inductor7/RConn1 -- Controlled Current Source3/RConn2 -- Variable Resistor3/LConn2 -- Resistor32/LConn1
  Simulink-PS Converter7/RConn1 -- Controlled Current Source3/RConn1
  Controlled Voltage Source2/RConn2 -- Electrical Reference1/LConn1 -- Voltage Sensor2/RConn2 -- Capacitor1/RConn1 -- Variable Resistor2/RConn1 -- Controlled Current Source2/LConn1
  Simulink-PS Converter3/RConn1 -- Controlled Voltage Source4/RConn1
  Simulink-PS Converter1/RConn1 -- Controlled Voltage Source2/RConn1
  Controlled Voltage Source1/RConn2 -- Electrical Reference/LConn1 -- Voltage Sensor/RConn2 -- Capacitor/RConn1 -- Controlled Current Source1/LConn1 -- Variable Resistor1/RConn1
  Simulink-PS Converter/RConn1 -- Controlled Voltage Source1/RConn1
  Resistor/RConn1 -- Inductor/LConn1
  Resistor10/RConn1 -- Inductor7/LConn1
  Simulink-PS Converter4/RConn1 -- Controlled Current Source/RConn1
  Resistor5/RConn1 -- Inductor3/LConn1
  Simulink-PS Converter2/RConn1 -- Controlled Voltage Source3/RConn1
  Simulink-PS Converter5/RConn1 -- Controlled Current Source1/RConn1
  Controlled Current Source2/RConn1 -- Simulink-PS Converter6/RConn1
  Current Sensor/LConn1 -- Controlled Voltage Source2/LConn1
  Current Sensor/RConn2 -- Resistor3/LConn1
  Current Sensor1/RConn2 -- Resistor10/LConn1
  Current Sensor1/LConn1 -- Controlled Voltage Source4/LConn1
  Current Sensor2/RConn2 -- Resistor5/LConn1
  Current Sensor2/LConn1 -- Controlled Voltage Source3/LConn1
  Current Sensor3/RConn2 -- Resistor/LConn1
  Current Sensor3/LConn1 -- Controlled Voltage Source1/LConn1 -- Solver Configuration/RConn1
  Current Sensor3/RConn1 -- PS-Simulink Converter/LConn1
  Current Sensor2/RConn1 -- PS-Simulink Converter1/LConn1
  PS-Simulink Converter2/LConn1 -- Current Sensor/RConn1
  PS-Simulink Converter3/LConn1 -- Current Sensor1/RConn1
  Variable Resistor1/LConn1 -- Simulink-PS Converter8/RConn1
  Variable Resistor2/LConn1 -- Simulink-PS Converter9/RConn1
  Variable Resistor3/LConn1 -- Simulink-PS Converter10/RConn1
  Simulink-PS Converter11/RConn1 -- Variable Resistor/LConn1
  Capacitor7/RConn1 -- Voltage Sensor6/RConn2 -- Controlled Voltage Source8/RConn2 -- Electrical Reference7/LConn1 -- Variable Resistor7/RConn1 -- Controlled Current Source7/LConn1
  Inductor32/LConn1 -- Resistor13/LConn1 -- Inductor12/RConn1 -- Voltage Sensor7/LConn1 -- Capacitor6/LConn1 -- Inductor11/RConn1 -- Controlled Current Source4/RConn2 -- Variable Resistor4/LConn2 -- Resistor43/RConn1
  Controlled Voltage Source7/RConn2 -- Electrical Reference6/LConn1 -- Voltage Sensor7/RConn2 -- Capacitor6/RConn1 -- Variable Resistor4/RConn1 -- Controlled Current Source4/LConn1
  Capacitor7/LConn1 -- Voltage Sensor6/LConn1 -- Inductor15/RConn1 -- Controlled Current Source7/RConn2 -- Inductor14/RConn1 -- Inductor13/RConn1 -- Variable Resistor7/LConn2
  Controlled Voltage Source6/RConn2 -- Electrical Reference5/LConn1 -- Voltage Sensor5/RConn2 -- Capacitor5/RConn1 -- Variable Resistor6/RConn1 -- Controlled Current Source6/LConn1
  Inductor8/RConn1 -- Capacitor4/LConn1 -- Voltage Sensor4/LConn1 -- Resistor15/LConn1 -- Resistor6/LConn1 -- Variable Resistor5/LConn2 -- Controlled Current Source5/RConn2
  Resistor14/LConn1 -- Inductor9/RConn1 -- Variable Resistor6/LConn2 -- Controlled Current Source6/RConn2 -- Voltage Sensor5/LConn1 -- Capacitor5/LConn1 -- Inductor10/RConn1
  Controlled Voltage Source5/RConn2 -- Variable Resistor5/RConn1 -- Controlled Current Source5/LConn1 -- Electrical Reference4/LConn1 -- Voltage Sensor4/RConn2 -- Capacitor4/RConn1
  Current Sensor7/LConn1 -- Controlled Voltage Source5/LConn1
  Current Sensor4/RConn2 -- Resistor11/LConn1
  Variable Resistor7/LConn1 -- Simulink-PS Converter14/RConn1
  Simulink-PS Converter12/RConn1 -- Controlled Voltage Source5/RConn1
  Current Sensor6/LConn1 -- Controlled Voltage Source7/LConn1
  PS-Simulink Converter7/LConn1 -- Current Sensor5/RConn1
  Simulink-PS Converter15/RConn1 -- Variable Resistor4/LConn1
  Variable Resistor6/LConn1 -- Simulink-PS Converter23/RConn1
  PS-Simulink Converter6/LConn1 -- Current Sensor4/RConn1
  Resistor1/RConn1 -- Inductor8/LConn1
  Simulink-PS Converter17/RConn1 -- Controlled Voltage Source8/RConn1
  Resistor12/RConn1 -- Inductor11/LConn1
  Current Sensor6/RConn2 -- Resistor12/LConn1
  Resistor4/RConn1 -- Inductor15/LConn1
  Resistor11/RConn1 -- Inductor10/LConn1
  Current Sensor4/LConn1 -- Controlled Voltage Source6/LConn1
  Current Sensor7/RConn1 -- PS-Simulink Converter4/LConn1
  Controlled Current Source6/RConn1 -- Simulink-PS Converter20/RConn1
  Simulink-PS Converter19/RConn1 -- Controlled Current Source5/RConn1
  Variable Resistor5/LConn1 -- Simulink-PS Converter22/RConn1
  Current Sensor7/RConn2 -- Resistor1/LConn1
  Simulink-PS Converter21/RConn1 -- Controlled Current Source7/RConn1
  Current Sensor5/LConn1 -- Controlled Voltage Source8/LConn1
  Current Sensor6/RConn1 -- PS-Simulink Converter5/LConn1
  Simulink-PS Converter16/RConn1 -- Controlled Voltage Source7/RConn1
  Simulink-PS Converter13/RConn1 -- Controlled Voltage Source6/RConn1
  Current Sensor5/RConn2 -- Resistor4/LConn1
  Simulink-PS Converter18/RConn1 -- Controlled Current Source4/RConn1
  Controlled Current Source8/LConn1 -- Controlled Voltage Source11/RConn2 -- Electrical Reference10/LConn1 -- Voltage Sensor11/RConn2 -- Capacitor10/RConn1 -- Variable Resistor8/RConn1
  Inductor17/RConn1 -- Voltage Sensor11/LConn1 -- Capacitor10/LConn1 -- Controlled Current Source8/RConn2 -- Inductor18/RConn1 -- Resistor19/LConn1 -- Variable Resistor8/LConn2
  Capacitor11/RConn1 -- Voltage Sensor10/RConn2 -- Controlled Voltage Source12/RConn2 -- Electrical Reference11/LConn1 -- Controlled Current Source11/LConn1 -- Variable Resistor11/RConn1
  Inductor33/RConn1 -- Resistor21/LConn1 -- Resistor23/LConn1 -- Voltage Sensor8/LConn1 -- Capacitor8/LConn1 -- Inductor22/RConn1 -- Controlled Current Source9/RConn2 -- Variable Resistor9/LConn2 -- Inductor43/LConn1
  Inductor23/RConn1 -- Variable Resistor10/LConn2 -- Controlled Current Source10/RConn2 -- Voltage Sensor9/LConn1 -- Capacitor9/LConn1 -- Inductor16/RConn1 -- Resistor20/LConn1
  Capacitor11/LConn1 -- Voltage Sensor10/LConn1 -- Inductor21/RConn1 -- Inductor19/RConn1 -- Inductor20/RConn1 -- Variable Resistor11/LConn2 -- Controlled Current Source11/RConn2
  Electrical Reference8/LConn1 -- Controlled Voltage Source9/RConn2 -- Voltage Sensor8/RConn2 -- Capacitor8/RConn1 -- Controlled Current Source9/LConn1 -- Variable Resistor9/RConn1
  Capacitor9/RConn1 -- Voltage Sensor9/RConn2 -- Controlled Voltage Source10/RConn2 -- Electrical Reference9/LConn1 -- Variable Resistor10/RConn1 -- Controlled Current Source10/LConn1
  Current Sensor11/RConn2 -- Resistor16/LConn1
  Current Sensor10/RConn2 -- Resistor18/LConn1
  Simulink-PS Converter25/RConn1 -- Controlled Voltage Source10/RConn1
  Simulink-PS Converter30/RConn1 -- Controlled Current Source8/RConn1
  Controlled Current Source10/RConn1 -- Simulink-PS Converter32/RConn1
  Variable Resistor11/LConn1 -- Simulink-PS Converter26/RConn1
  Current Sensor11/LConn1 -- Controlled Voltage Source9/LConn1
  Simulink-PS Converter24/RConn1 -- Controlled Voltage Source9/RConn1
  Current Sensor8/LConn1 -- Controlled Voltage Source10/LConn1
  Current Sensor10/RConn1 -- PS-Simulink Converter9/LConn1
  PS-Simulink Converter10/LConn1 -- Current Sensor8/RConn1
  Simulink-PS Converter33/RConn1 -- Controlled Current Source11/RConn1
  Current Sensor9/LConn1 -- Controlled Voltage Source12/LConn1
  PS-Simulink Converter11/LConn1 -- Current Sensor9/RConn1
  Variable Resistor10/LConn1 -- Simulink-PS Converter35/RConn1
  Simulink-PS Converter27/RConn1 -- Variable Resistor8/LConn1
  Resistor17/RConn1 -- Inductor16/LConn1
  Current Sensor11/RConn1 -- PS-Simulink Converter8/LConn1
  Current Sensor10/LConn1 -- Controlled Voltage Source11/LConn1
  Variable Resistor9/LConn1 -- Simulink-PS Converter34/RConn1
  Simulink-PS Converter28/RConn1 -- Controlled Voltage Source11/RConn1
  Current Sensor8/RConn2 -- Resistor17/LConn1
  Resistor16/RConn1 -- Inductor22/LConn1
  Current Sensor9/RConn2 -- Resistor22/LConn1
  Simulink-PS Converter29/RConn1 -- Controlled Voltage Source12/RConn1
  Resistor22/RConn1 -- Inductor21/LConn1
  Resistor18/RConn1 -- Inductor17/LConn1
  Simulink-PS Converter31/RConn1 -- Controlled Current Source9/RConn1
  Controlled Current Source12/LConn1 -- Controlled Voltage Source15/RConn2 -- Electrical Reference14/LConn1 -- Voltage Sensor15/RConn2 -- Capacitor14/RConn1 -- Variable Resistor12/RConn1
  Inductor25/RConn1 -- Voltage Sensor15/LConn1 -- Capacitor14/LConn1 -- Controlled Current Source12/RConn2 -- Inductor26/RConn1 -- Resistor27/LConn1 -- Variable Resistor12/LConn2
  Capacitor15/RConn1 -- Voltage Sensor14/RConn2 -- Controlled Voltage Source16/RConn2 -- Electrical Reference15/LConn1 -- Controlled Current Source15/LConn1 -- Variable Resistor15/RConn1
  Inductor30/RConn1 -- Voltage Sensor12/LConn1 -- Capacitor12/LConn1 -- Resistor29/LConn1 -- Resistor31/LConn1 -- Variable Resistor13/LConn2 -- Controlled Current Source13/RConn2
  Inductor31/RConn1 -- Resistor33/LConn1 -- Inductor42/RConn1 -- Resistor28/LConn1 -- Variable Resistor14/LConn2 -- Voltage Sensor13/LConn1 -- Capacitor13/LConn1 -- Inductor24/RConn1 -- Controlled Current Source14/RConn2
  Capacitor15/LConn1 -- Voltage Sensor14/LConn1 -- Inductor29/RConn1 -- Inductor27/RConn1 -- Inductor28/RConn1 -- Variable Resistor15/LConn2 -- Controlled Current Source15/RConn2
  Electrical Reference12/LConn1 -- Controlled Current Source13/LConn1 -- Variable Resistor13/RConn1 -- Controlled Voltage Source13/RConn2 -- Voltage Sensor12/RConn2 -- Capacitor12/RConn1
  Capacitor13/RConn1 -- Voltage Sensor13/RConn2 -- Controlled Voltage Source14/RConn2 -- Electrical Reference13/LConn1 -- Variable Resistor14/RConn1 -- Controlled Current Source14/LConn1
  Current Sensor15/RConn2 -- Resistor24/LConn1
  Current Sensor14/RConn2 -- Resistor26/LConn1
  Simulink-PS Converter37/RConn1 -- Controlled Voltage Source14/RConn1
  Simulink-PS Converter42/RConn1 -- Controlled Current Source12/RConn1
  Controlled Current Source14/RConn1 -- Simulink-PS Converter44/RConn1
  Variable Resistor15/LConn1 -- Simulink-PS Converter38/RConn1
  Current Sensor15/LConn1 -- Controlled Voltage Source13/LConn1
  Simulink-PS Converter36/RConn1 -- Controlled Voltage Source13/RConn1
  Current Sensor12/LConn1 -- Controlled Voltage Source14/LConn1
  Current Sensor14/RConn1 -- PS-Simulink Converter13/LConn1
  PS-Simulink Converter14/LConn1 -- Current Sensor12/RConn1
  Simulink-PS Converter45/RConn1 -- Controlled Current Source15/RConn1
  Current Sensor13/LConn1 -- Controlled Voltage Source16/LConn1
  PS-Simulink Converter15/LConn1 -- Current Sensor13/RConn1
  Variable Resistor14/LConn1 -- Simulink-PS Converter47/RConn1
  Simulink-PS Converter39/RConn1 -- Variable Resistor12/LConn1
  Resistor25/RConn1 -- Inductor24/LConn1
  Current Sensor15/RConn1 -- PS-Simulink Converter12/LConn1
  Current Sensor14/LConn1 -- Controlled Voltage Source15/LConn1
  Variable Resistor13/LConn1 -- Simulink-PS Converter46/RConn1
  Simulink-PS Converter40/RConn1 -- Controlled Voltage Source15/RConn1
  Current Sensor12/RConn2 -- Resistor25/LConn1
  Resistor24/RConn1 -- Inductor30/LConn1
  Current Sensor13/RConn2 -- Resistor30/LConn1
  Simulink-PS Converter41/RConn1 -- Controlled Voltage Source16/RConn1
  Resistor30/RConn1 -- Inductor29/LConn1
  Resistor26/RConn1 -- Inductor25/LConn1
  Simulink-PS Converter43/RConn1 -- Controlled Current Source13/RConn1
  Current Sensor19/LConn1 -- Inductor5/LConn1
  Resistor7/RConn1 -- Current Sensor19/RConn2
  Resistor2/RConn1 -- Current Sensor18/LConn1
  Inductor1/LConn1 -- Current Sensor18/RConn2
  PS-Simulink Converter17/LConn1 -- Current Sensor18/RConn1
  PS-Simulink Converter19/LConn1 -- Current Sensor19/RConn1
  Inductor9/LConn1 -- Current Sensor20/RConn2
  PS-Simulink Converter20/LConn1 -- Current Sensor20/RConn1
  Current Sensor20/LConn1 -- Resistor6/RConn1
  PS-Simulink Converter21/LConn1 -- Current Sensor21/RConn1
  PS-Simulink Converter22/LConn1 -- Current Sensor22/RConn1
  Current Sensor22/LConn1 -- Resistor14/RConn1
  Current Sensor22/RConn2 -- Inductor14/LConn1
  Current Sensor23/LConn1 -- Inductor13/LConn1
  PS-Simulink Converter23/LConn1 -- Current Sensor23/RConn1
  Current Sensor23/RConn2 -- Resistor13/RConn1
  Current Sensor28/LConn1 -- Resistor23/RConn1
  PS-Simulink Converter24/LConn1 -- Current Sensor28/RConn1
  Current Sensor28/RConn2 -- Inductor23/LConn1
  PS-Simulink Converter25/LConn1 -- Current Sensor30/RConn1
  Inductor20/LConn1 -- Current Sensor30/RConn2
  Resistor20/RConn1 -- Current Sensor30/LConn1
  PS-Simulink Converter26/LConn1 -- Current Sensor29/RConn1
  Inductor19/LConn1 -- Current Sensor31/LConn1
  Resistor19/RConn1 -- Current Sensor31/RConn2
  PS-Simulink Converter27/LConn1 -- Current Sensor31/RConn1
  Current Sensor33/RConn2 -- Inductor31/LConn1
  PS-Simulink Converter28/LConn1 -- Current Sensor33/RConn1
  Current Sensor33/LConn1 -- Resistor31/RConn1
  Inductor27/LConn1 -- Current Sensor35/LConn1
  PS-Simulink Converter29/LConn1 -- Current Sensor35/RConn1
  Resistor27/RConn1 -- Current Sensor35/RConn2
  PS-Simulink Converter30/LConn1 -- Current Sensor32/RConn1
  PS-Simulink Converter31/LConn1 -- Current Sensor34/RConn1
  Resistor28/RConn1 -- Current Sensor34/LConn1
  Current Sensor27/LConn1 -- Resistor42/LConn1
  PS-Simulink Converter33/LConn1 -- Current Sensor27/RConn1
  Inductor42/LConn1 -- Current Sensor27/RConn2
  PS-Simulink Converter35/LConn1 -- Current Sensor24/RConn1
  Voltage Sensor/RConn1 -- PS-Simulink Converter36/LConn1
  Voltage Sensor1/RConn1 -- PS-Simulink Converter37/LConn1
  Voltage Sensor2/RConn1 -- PS-Simulink Converter38/LConn1
  Voltage Sensor3/RConn1 -- PS-Simulink Converter39/LConn1
  Voltage Sensor4/RConn1 -- PS-Simulink Converter40/LConn1
  Voltage Sensor5/RConn1 -- PS-Simulink Converter41/LConn1
  Voltage Sensor6/RConn1 -- PS-Simulink Converter42/LConn1
  Voltage Sensor7/RConn1 -- PS-Simulink Converter43/LConn1
  Voltage Sensor8/RConn1 -- PS-Simulink Converter44/LConn1
  Voltage Sensor9/RConn1 -- PS-Simulink Converter45/LConn1
  Voltage Sensor10/RConn1 -- PS-Simulink Converter46/LConn1
  Voltage Sensor11/RConn1 -- PS-Simulink Converter47/LConn1
  Voltage Sensor12/RConn1 -- PS-Simulink Converter48/LConn1
  Voltage Sensor13/RConn1 -- PS-Simulink Converter49/LConn1
  Voltage Sensor14/RConn1 -- PS-Simulink Converter50/LConn1
  Voltage Sensor15/RConn1 -- PS-Simulink Converter51/LConn1
  Current Sensor16/RConn1 -- PS-Simulink Converter16/LConn1
  Resistor8/RConn1 -- Current Sensor17/LConn1
  Current Sensor17/RConn2 -- Inductor6/LConn1
  PS-Simulink Converter18/LConn1 -- Current Sensor17/RConn1
  Current Sensor34/RConn2 -- Inductor28/LConn1
  PS-Simulink Converter34/LConn1 -- Current Sensor26/RConn1
  PS-Simulink Converter32/LConn1 -- Current Sensor25/RConn1
  Resistor9/RConn1 -- Current Sensor16/LConn1
  Current Sensor16/RConn2 -- Inductor4/LConn1
  Resistor15/RConn1 -- Current Sensor21/LConn1
  Current Sensor21/RConn2 -- Inductor12/LConn1
  Resistor21/RConn1 -- Current Sensor29/LConn1
  Inductor18/LConn1 -- Current Sensor29/RConn2
  Resistor29/RConn1 -- Current Sensor32/LConn1
  Current Sensor32/RConn2 -- Inductor26/LConn1
  Resistor32/RConn1 -- Current Sensor25/LConn1
  Inductor32/RConn1 -- Current Sensor25/RConn2
  Resistor43/LConn1 -- Current Sensor26/LConn1
  Current Sensor26/RConn2 -- Inductor43/RConn1
  Resistor33/RConn1 -- Current Sensor24/RConn2
  Current Sensor24/LConn1 -- Inductor33/LConn1
